simulink model "Task5"  (R2022a)
settings: Solver=FixedStepAuto  StartTime=0.0  StopTime=10.0  FixedStep=0.001  RelTol=1e-3
undefined symbols (not defined in the file): k1, k2
settings Model: Creator=Family  LastModifiedBy=Family

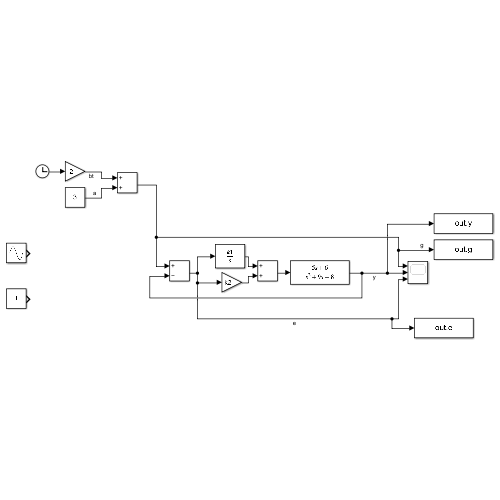
[thumbnail: Simulink's stored preview of the top-level diagram]
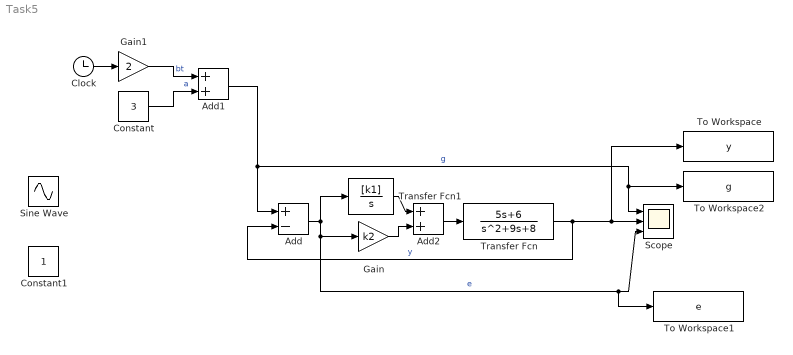
== system Task5 ==
  Add : Sum  Inputs=+-
  Add1 : Sum
  Add2 : Sum
  Clock : Clock
  Constant : Constant  Value=3  SampleTime=-1
  Constant1 : Constant  SampleTime=-1
  Gain : Gain  Gain=k2
  Gain1 : Gain  Gain=2
  Scope : Scope  NumInputPorts=3
  Sine Wave : Sin  Amplitude=2  Phase=2  SampleTime=0
  To Workspace : ToWorkspace  VariableName=y  SaveFormat=Timeseries  SampleTime=-1
  To Workspace1 : ToWorkspace  VariableName=e  SaveFormat=Timeseries  SampleTime=-1
  To Workspace2 : ToWorkspace  VariableName=g  SaveFormat=Timeseries  SampleTime=-1
  Transfer Fcn : TransferFcn  Numerator=[5 6]  Denominator=[1 9 8]
  Transfer Fcn1 : TransferFcn  Numerator=[k1]  Denominator=[1 0]
  wires:
  Transfer Fcn/1 -> Add/2, To Workspace/1, Scope/2  "y"
  Add/1 -> Transfer Fcn1/1, Gain/1, To Workspace1/1, Scope/3  "e"
  Add1/1 -> Add/1, Scope/1, To Workspace2/1  "g"
  Clock/1 -> Gain1/1
  Gain1/1 -> Add1/1  "bt"
  Constant/1 -> Add1/2  "a"
  Add2/1 -> Transfer Fcn/1
  Transfer Fcn1/1 -> Add2/1
  Gain/1 -> Add2/2
